simulink model "discrete_kalman_filter"  (R2015b)
settings: Solver=VariableStepAuto  StartTime=0.0  StopTime=10.0  RelTol=1e-3
undefined symbols (not defined in the file or in its folder): A, b, g, I, k, KF_P0, KF_Q, KF_R, l, m
settings Model: Creator=mgreiff  LastModifiedBy=mgreiff

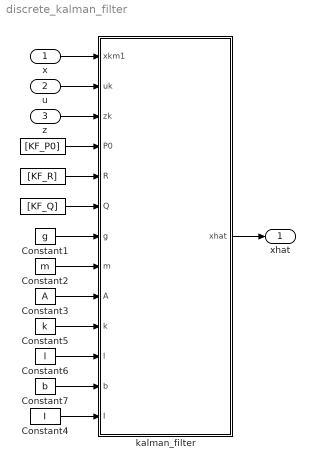
== system discrete_kalman_filter ==
  x : Inport  PortDimensions=12
  u : Inport  Port=2  PortDimensions=4
  z : Inport  Port=3  PortDimensions=7
  " " : Constant  Value=[KF_P0]
  "  " : Constant  Value=[KF_R]
  "   " : Constant  Value=[KF_Q]
  Constant1 : Constant  Value=g
  Constant2 : Constant  Value=m
  Constant3 : Constant  Value=A
  Constant4 : Constant  Value=I
  Constant5 : Constant  Value=k
  Constant6 : Constant  Value=l
  Constant7 : Constant  Value=b
  kalman_filter : MATLAB Function  TreatAsAtomicUnit=on
  xhat : Outport  PortDimensions=12
  wires:
  x/1 -> kalman_filter/1(xkm1)
  u/1 -> kalman_filter/2(uk)
  z/1 -> kalman_filter/3(zk)
  " "/1 -> kalman_filter/4(P0)
  "  "/1 -> kalman_filter/5(R)
  "   "/1 -> kalman_filter/6(Q)
  kalman_filter/1(xhat) -> xhat/1
  Constant3/1 -> kalman_filter/9(A)
  Constant2/1 -> kalman_filter/8(m)
  Constant1/1 -> kalman_filter/7(g)
  Constant4/1 -> kalman_filter/13(I)
  Constant5/1 -> kalman_filter/10(k)
  Constant6/1 -> kalman_filter/11(l)
  Constant7/1 -> kalman_filter/12(b)

== matlab function discrete_kalman_filter/kalman_filter ==
  data: xhat output; xkm1 input; uk input; zk input; P0 input; R input; Q input; g input; m input; A input; k input; l input; b input; I input
function xhat  = fcn(xkm1, uk, zk, P0, R, Q, g, m, A, k, l, b, I)
%#codegen
% xkm1  = [x,             uk = [e_z,         zk = [z,
%          y,                   e_phi,             dotx,
%          z,                   e_theta]           doty,
%          dotx,                                   dotz,
%          doty,                                   theta,
%          dotz,                                   phi]
%          phi,
%          theta,
%          dotphi,
%          dottheta]

persistent P

if isempty(P)
    P = P0;
end
%% Set up basic continuous-model dynamics, including PD

Ixx = I(1); Iyy=I(2); Izz = I(3);

Ac = zeros(12);
Ac(1:3,4:6) = eye(3);
Ac(4:6,4:6) = -diag(A)/m;
Ac(7:9,10:12) = eye(3);

Bc = zeros(12, 4);
Bc(6, :) = k;
Bc(10:12,:) = [0,-k*l/Ixx,0,k*l/Ixx;
              -k*l/Iyy,0,k*l/Iyy,0;
              -b/Izz,b/Izz,-b/Izz,b/Izz];
Bc = sqrt(m*g/k).*Bc;

Cc = zeros(7, 12);
Cc(1:7,3:9) = eye(7);

Dc = zeros(7, 4);

% contsys = ss(Ac,Bc,Cc,Dc);
% discsys = c2d(contsys, 0.01);
% [Ad, Bd, Cd, Dd] = ssdata(discsys);

Ad1 = [1.000000000000000                   0                   0   0.009973338094320                   0;
                       0   1.000000000000000                   0                   0   0.009973338094320;
                       0                   0   1.000000000000000                   0                   0;
                       0                   0                   0   0.994672362129102                   0;
                       0                   0                   0                   0   0.994672362129102;
                       0                   0                   0                   0                   0;
                       0                   0                   0                   0                   0;
                       0                   0                   0                   0                   0;
                       0                   0                   0                   0                   0;
                       0                   0                   0                   0                   0;
                       0                   0                   0                   0                   0;
                       0                   0                   0                   0                   0];

Ad2 = [                0 0 0 0    0;
                       0 0 0 0    0;
       0.009973338094320 0 0 0    0;
                       0 0 0 0    0;
                       0 0 0 0    0;
       0.994672362129102 0 0 0    0;
                       0 1 0 0 0.01;
                       0 0 1 0    0;
                       0 0 0 1    0;
                       0 0 0 0    1;
                       0 0 0 0    0;
                       0 0 0 0    0];
Ad3 = [0 0;
       0 0;
       0 0;
       0 0;
       0 0;
       0 0;
       0 0;
       0.01 0;
       0 0.01;
       0 0;
       1 0;
       0 1];

Ad = [Ad1, Ad2, Ad3];

Bd = [                 0                   0                   0                   0;
                       0                   0                   0                   0;
       0.000000184613134   0.000000184613134   0.000000184613134   0.000000184613134;
                       0                   0                   0                   0;
                       0                   0                   0                   0;
       0.000036889783298   0.000036889783298   0.000036889783298   0.000036889783298;
                       0  -0.000008569182785                   0   0.000008569182785;
      -0.000008569182785                   0   0.000008569182785                   0;
      -0.000000803881683   0.000000803881683  -0.000000803881683   0.000000803881683;
                       0  -0.001713836556980                   0   0.001713836556980;
      -0.001713836556980                   0   0.001713836556980                   0;
      -0.000160776336524   0.000160776336524  -0.000160776336524   0.000160776336524];
  
Cd = Cc;
% Predictor step
xf = Ad * xkm1 + Bd * uk;
Pf = Ad * P * Ad' + Q;

% Corrector step
K =  Pf * Cd' / (Cd * Pf * Cd'+ R);
xhat = xf + K * (zk - Cd * xf);
P = (eye(12) - K * Cd) * Pf;
